simulink model "wlan_phy_tx_pmd"  (Simulink 7.8)
settings: Solver=VariableStepDiscrete  SolverMode=SingleTasking  StartTime=0.0  StopTime=inf  RelTol=1e-3
PostLoadFcn:
  | wlan_phy_tx_init
InitFcn:
  | wlan_phy_tx_init
StartFcn:
  | wlan_phy_tx_init
undefined symbols (not defined in the file): gcbh, ht_preamble_rom, MAX_CP_LEN, MAX_DATA_BITS_PER_SYM_PERIOD, MAX_NCBPS, MAX_NUM_BYTES, MAX_NUM_SC, MAX_NUM_SYMS, mcs_rom_11ag, mcs_rom_11n, Mod_Constellation_16QAM, Mod_Constellation_64QAM, Mod_Constellation_BPSK, Mod_Constellation_QPSK, Preamble_IQ, Preamble_IQ_scaled, tx_sim, wlan_tx_interleave_rom, xlBlockLoadCallback, xlGetNormalizedPeriod
libraries: xbsIndex_r4 x1358, xbsEDKLib_r4 x1
(part 9 of 10)

== system wlan_phy_tx_pmd/PSDU Syms Gen/Puncture & Interleave/Interleaver Ctrl & Puncturing/Interleave Mapping ==
  Base Rate Sym : Inport
  Ind A : Inport  Port=2
  Ind B : Inport  Port=3
  Concat1 : xbsIndex_r4/Concat  num_inputs=2  dbl_ovrd=off  block_type=concat
  Concat2 : xbsIndex_r4/Concat  num_inputs=3  dbl_ovrd=off  block_type=concat
  Concat3 : xbsIndex_r4/Concat  num_inputs=3  dbl_ovrd=off  block_type=concat
  Constant8 : xbsIndex_r4/Constant  const=0  gui_display_data_type=Fixed-point  arith_type=Unsigned  n_bits=ceil(log2(MAX_NCBPS))  bin_pt=0  preci_type=Single  exp_width=8  frac_width=24  explicit_period=off  period=1  equ=P=C  opselect=C  inp2=PCIN>>17  opr=+  inp1=P  carry=CIN  dbl_ovrd=off  block_type=constant
  Constant9 : xbsIndex_r4/Constant  const=0  gui_display_data_type=Boolean  arith_type=Boolean  n_bits=2  bin_pt=0  preci_type=Single  exp_width=8  frac_width=24  explicit_period=off  period=1  equ=P=C  opselect=C  inp2=PCIN>>17  opr=+  inp1=P  carry=CIN  dbl_ovrd=off  block_type=constant
  Inverter : xbsIndex_r4/Inverter  en=off  latency=0  dbl_ovrd=off  block_type=inv
  Logical : xbsIndex_r4/Logical  logical_function=AND  inputs=2  en=off  latency=0  precision=Full  arith_type=Unsigned  n_bits=16  bin_pt=0  align_bp=on  dbl_ovrd=off  block_type=logical
  Logical1 : xbsIndex_r4/Logical  logical_function=AND  inputs=2  en=off  latency=0  precision=Full  arith_type=Unsigned  n_bits=16  bin_pt=0  align_bp=on  dbl_ovrd=off  block_type=logical
  Map ROM : xbsIndex_r4/Dual Port RAM  depth=length(wlan_tx_interleave_rom)  initVector=wlan_tx_interleave_rom  distributed_mem=Block RAM  init_a=0  init_b=0  rst_a=off  rst_b=off  en_a=off  en_b=off  latency=1  write_mode_A=Read After Write  write_mode_B=Read After Write  dbl_ovrd=off  optimize=Area  block_type=dpram
  Addr A : Outport
  Addr B : Outport  Port=2
  wires:
  Base Rate Sym/1 -> Inverter/1
  Inverter/1 -> Logical/2, Concat1/1, Concat1/2
  Logical/1 -> Concat2/1, Concat3/1
  Logical1/1 -> Concat2/2, Concat3/2
  Ind A/1 -> Concat2/3
  [Tx_PHY_Mode_11n] -> Logical/1
  Concat2/1 -> Map ROM/1
  Ind B/1 -> Concat3/3
  Concat3/1 -> Map ROM/4
  Constant8/1 -> Map ROM/2, Map ROM/5
  Constant9/1 -> Map ROM/3, Map ROM/6
  Map ROM/1 -> Addr A/1
  Map ROM/2 -> Addr B/1
  [OFDM_TX_DATA_Mod_Sel] -> Logical1/2
  Concat1/1 -> Logical1/1

== system wlan_phy_tx_pmd/PSDU Syms Gen/Puncture & Interleave/Interleaver Ctrl & Puncturing/Puncturing ==
  Code Rate : Inport
  Reset : Inport  Port=2
  En : Inport  Port=3
  Inverter : xbsIndex_r4/Inverter  en=off  latency=0  dbl_ovrd=off  block_type=inv
  Inverter1 : xbsIndex_r4/Inverter  en=off  latency=0  dbl_ovrd=off  block_type=inv
  Logical : xbsIndex_r4/Logical  logical_function=AND  inputs=2  en=off  latency=0  precision=Full  arith_type=Unsigned  n_bits=16  bin_pt=0  align_bp=on  dbl_ovrd=off  block_type=logical
  Logical1 : xbsIndex_r4/Logical  logical_function=AND  inputs=2  en=off  latency=0  precision=Full  arith_type=Unsigned  n_bits=16  bin_pt=0  align_bp=on  dbl_ovrd=off  block_type=logical
  Mux1 : xbsIndex_r4/Mux  inputs=4  en=off  latency=0  precision=Full  arith_type=Unsigned  n_bits=16  bin_pt=14  quantization=Truncate  overflow=Wrap  dbl_ovrd=off  block_type=mux
  Mux3 : xbsIndex_r4/Mux  inputs=4  en=off  latency=0  precision=Full  arith_type=Unsigned  n_bits=16  bin_pt=14  quantization=Truncate  overflow=Wrap  dbl_ovrd=off  block_type=mux
  Mux4 : xbsIndex_r4/Mux  inputs=4  en=off  latency=0  precision=Full  arith_type=Unsigned  n_bits=16  bin_pt=14  quantization=Truncate  overflow=Wrap  dbl_ovrd=off  block_type=mux
  Rate 1/2 : Subsystem
  Rate 2/3 : Subsystem
  Rate 3/4 : Subsystem
  Rate 5/6 : Subsystem
  Index Inc : Outport
  Wr A : Outport  Port=2
  Wr B : Outport  Port=3
  wires:
  Mux3/1 -> Inverter/1
  Rate 1/2/1(Ind Inc) -> [R12_INC_A]
  Rate 1/2/2(Skip A) -> [R12_SKIP_A]
  Rate 1/2/3(Skip B) -> [R12_SKIP_B]
  Rate 2/3/1(Ind Inc) -> [R23_INC_A]
  Rate 2/3/2(Skip A) -> [R23_SKIP_A]
  Rate 2/3/3(Skip B) -> [R23_SKIP_B]
  Rate 3/4/1(Ind Inc) -> [R34_INC_A]
  Rate 3/4/2(Skip A) -> [R34_SKIP_A]
  Rate 3/4/3(Skip B) -> [R34_SKIP_B]
  [R12_SKIP_A] -> Mux3/2
  [R23_SKIP_A] -> Mux3/3
  [R34_SKIP_A] -> Mux3/4
  Mux1/1 -> Inverter1/1
  [R12_SKIP_B] -> Mux1/2
  [R23_SKIP_B] -> Mux1/3
  [R34_SKIP_B] -> Mux1/4
  [R12_INC_A] -> Mux4/2
  [R23_INC_A] -> Mux4/3
  [R34_INC_A] -> Mux4/4
  [R56_INC_A] -> Mux4/5
  [R56_SKIP_A] -> Mux3/5
  Rate 5/6/1(Ind Inc) -> [R56_INC_A]
  Rate 5/6/2(Skip A) -> [R56_SKIP_A]
  Rate 5/6/3(Skip B) -> [R56_SKIP_B]
  [R56_SKIP_B] -> Mux1/5
  Code Rate/1 -> Mux4/1, Mux3/1, Mux1/1
  Mux4/1 -> Index Inc/1
  Inverter/1 -> Logical/1
  Inverter1/1 -> Logical1/1
  Reset/1 -> Rate 1/2/1(Rst), Rate 2/3/1(Rst), Rate 3/4/1(Rst), Rate 5/6/1(Rst)
  En/1 -> Rate 1/2/2(En), Rate 2/3/2(En), Rate 3/4/2(En), Rate 5/6/2(En), Logical1/2, Logical/2
  Logical/1 -> Wr A/1
  Logical1/1 -> Wr B/1

== system wlan_phy_tx_pmd/PSDU Syms Gen/Puncture & Interleave/Interleaver Ctrl & Puncturing/negedge ==
  D : Inport
  Delay : xbsIndex_r4/Delay  rst=off  infoeditControl=Selection of Reset will increase slice count due to use of real FFs and instead of SRLs  en=off  latency=1  dbl_ovrd=off  reg_retiming=off  block_type=delay
      settings: infoedit=Hardware notes: A delay line is a chain, each link of which is an SRL16 followed by a flip-flop. If register retiming is enabled, the delay line is a chain of flip-flops.  xl_area=[1 1 0 0 0 0 0]  block_version=VER_STRING_GOES_HERE
  Inverter : xbsIndex_r4/Inverter  en=off  latency=0  dbl_ovrd=off  block_type=inv
      settings: xl_area=[0 0 0 0 0 0 0]  block_version=VER_STRING_GOES_HERE
  Logical1 : xbsIndex_r4/Logical  logical_function=AND  inputs=2  en=off  latency=0  precision=Full  arith_type=Unsigned  n_bits=8  bin_pt=2  align_bp=on  dbl_ovrd=off  block_type=logical
      settings: xl_area=[1 0 0 1 0 0 0]  block_version=VER_STRING_GOES_HERE
  Q : Outport
  wires:
  D/1 -> Delay/1, Inverter/1
  Logical1/1 -> Q/1
  Delay/1 -> Logical1/1
  Inverter/1 -> Logical1/2

== system wlan_phy_tx_pmd/PSDU Syms Gen/Puncture & Interleave/Mem Sel/S-R Latch1 ==
  S : Inport
  R : Inport  Port=2
  Constant1 : xbsIndex_r4/Constant  const=1  gui_display_data_type=Fixed-point  arith_type=Boolean  n_bits=1  bin_pt=0  preci_type=Single  exp_width=8  frac_width=24  explicit_period=off  period=1  equ=P=C  opselect=C  inp2=PCIN>>17  opr=+  inp1=P  carry=CIN  dbl_ovrd=off  block_type=constant
      settings: block_version=VER_STRING_GOES_HERE
  Convert1 : xbsIndex_r4/Convert  gui_display_data_type=Boolean  arith_type=Boolean  n_bits=1  bin_pt=0  float_type=Single  exp_bits=8  fraction_bits=24  quantization=Truncate  overflow=Wrap  en=off  latency=0  dbl_ovrd=off  pipeline=off  block_type=convert
  Convert2 : xbsIndex_r4/Convert  gui_display_data_type=Boolean  arith_type=Boolean  n_bits=1  bin_pt=0  float_type=Single  exp_bits=8  fraction_bits=24  quantization=Truncate  overflow=Wrap  en=off  latency=0  dbl_ovrd=off  pipeline=off  block_type=convert
  Register2 : xbsIndex_r4/Register  init=0  rst=on  en=on  dbl_ovrd=off  block_type=register
      settings: xl_area=[1 1 0 0 0 0 0]  block_version=VER_STRING_GOES_HERE
  Q : Outport
  wires:
  Convert2/1 -> Register2/3
  Convert1/1 -> Register2/2
  Constant1/1 -> Register2/1
  R/1 -> Convert1/1
  Register2/1 -> Q/1
  S/1 -> Convert2/1

== system wlan_phy_tx_pmd/Start Ctrl/Tx Active Debug Signal/Dly/S-R Latch1 ==
  S : Inport
  R : Inport  Port=2
  Constant1 : xbsIndex_r4/Constant  const=1  gui_display_data_type=Fixed-point  arith_type=Unsigned  n_bits=1  bin_pt=0  preci_type=Single  exp_width=8  frac_width=24  explicit_period=off  period=1  equ=P=C  opselect=C  inp2=PCIN>>17  opr=+  inp1=P  carry=CIN  dbl_ovrd=off  block_type=constant
      settings: block_version=VER_STRING_GOES_HERE
  Convert1 : xbsIndex_r4/Convert  gui_display_data_type=Boolean  arith_type=Boolean  n_bits=1  bin_pt=0  float_type=Single  exp_bits=8  fraction_bits=24  quantization=Truncate  overflow=Wrap  en=off  latency=0  dbl_ovrd=off  pipeline=off  block_type=convert
  Convert2 : xbsIndex_r4/Convert  gui_display_data_type=Boolean  arith_type=Boolean  n_bits=1  bin_pt=0  float_type=Single  exp_bits=8  fraction_bits=24  quantization=Truncate  overflow=Wrap  en=off  latency=0  dbl_ovrd=off  pipeline=off  block_type=convert
  Register2 : xbsIndex_r4/Register  init=0  rst=on  en=on  dbl_ovrd=off  block_type=register
      settings: xl_area=[1 1 0 0 0 0 0]  block_version=VER_STRING_GOES_HERE
  Q : Outport
  wires:
  Convert2/1 -> Register2/3
  Convert1/1 -> Register2/2
  Constant1/1 -> Register2/1
  R/1 -> Convert1/1
  Register2/1 -> Q/1
  S/1 -> Convert2/1

== system wlan_phy_tx_pmd/Start Ctrl/Tx Active Debug Signal/Dly/S-R Latch2 ==
  S : Inport
  R : Inport  Port=2
  Constant1 : xbsIndex_r4/Constant  const=1  gui_display_data_type=Fixed-point  arith_type=Unsigned  n_bits=1  bin_pt=0  preci_type=Single  exp_width=8  frac_width=24  explicit_period=off  period=1  equ=P=C  opselect=C  inp2=PCIN>>17  opr=+  inp1=P  carry=CIN  dbl_ovrd=off  block_type=constant
      settings: block_version=VER_STRING_GOES_HERE
  Convert1 : xbsIndex_r4/Convert  gui_display_data_type=Boolean  arith_type=Boolean  n_bits=1  bin_pt=0  float_type=Single  exp_bits=8  fraction_bits=24  quantization=Truncate  overflow=Wrap  en=off  latency=0  dbl_ovrd=off  pipeline=off  block_type=convert
  Convert2 : xbsIndex_r4/Convert  gui_display_data_type=Boolean  arith_type=Boolean  n_bits=1  bin_pt=0  float_type=Single  exp_bits=8  fraction_bits=24  quantization=Truncate  overflow=Wrap  en=off  latency=0  dbl_ovrd=off  pipeline=off  block_type=convert
  Register2 : xbsIndex_r4/Register  init=0  rst=on  en=on  dbl_ovrd=off  block_type=register
      settings: xl_area=[1 1 0 0 0 0 0]  block_version=VER_STRING_GOES_HERE
  Q : Outport
  wires:
  S/1 -> Convert2/1
  Register2/1 -> Q/1
  R/1 -> Convert1/1
  Constant1/1 -> Register2/1
  Convert1/1 -> Register2/2
  Convert2/1 -> Register2/3

== system wlan_phy_tx_pmd/PSDU Syms Gen/Modulate/Control & Pilots/Pilot Gen/Pilot Selection ==
  note: All PHY modes:
      | -Pilot tones in subcarriers [-21,-7,7,21]
      | -Subcarriers [-7,-21] are x_ind [57,43]
      | -One pilot per OFDM sybmol is opposite sign of other 3
      |
      | 11a/g:
      | -Opposite sign always in subcarrier 21
      |
      | 11n/ac:
      | -Syms 0:4: Same as a/g
      | -Syms 5:6: No pilot tones in HT-STF, HT-LTF
      | -Syms 7:N: Opposite sign pilot rotates across 4 subcarriers sequentially:
      |    7: 21
      |    8: 7
      |    9: -21
      |    10: -7
      |     ...
      | Logic uses 2LSB of sym index to select current negative pilot subcarrier
  sc_ind : Inport
  Shift : Inport  Port=2
  Constant1 : xbsIndex_r4/Constant  const=21  gui_display_data_type=Fixed-point  arith_type=Unsigned  n_bits=6  bin_pt=0  preci_type=Single  exp_width=8  frac_width=24  explicit_period=off  period=8  equ=P=C  opselect=C  inp2=PCIN>>17  opr=+  inp1=P  carry=CIN  dbl_ovrd=off  block_type=constant
  Constant2 : xbsIndex_r4/Constant  const=7  gui_display_data_type=Fixed-point  arith_type=Unsigned  n_bits=6  bin_pt=0  preci_type=Single  exp_width=8  frac_width=24  explicit_period=off  period=8  equ=P=C  opselect=C  inp2=PCIN>>17  opr=+  inp1=P  carry=CIN  dbl_ovrd=off  block_type=constant
  Constant3 : xbsIndex_r4/Constant  const=64-7  gui_display_data_type=Fixed-point  arith_type=Unsigned  n_bits=6  bin_pt=0  preci_type=Single  exp_width=8  frac_width=24  explicit_period=off  period=8  equ=P=C  opselect=C  inp2=PCIN>>17  opr=+  inp1=P  carry=CIN  dbl_ovrd=off  block_type=constant
  Constant4 : xbsIndex_r4/Constant  const=64-21  gui_display_data_type=Fixed-point  arith_type=Unsigned  n_bits=6  bin_pt=0  preci_type=Single  exp_width=8  frac_width=24  explicit_period=off  period=8  equ=P=C  opselect=C  inp2=PCIN>>17  opr=+  inp1=P  carry=CIN  dbl_ovrd=off  block_type=constant
  Logical1 : xbsIndex_r4/Logical  logical_function=OR  inputs=4  en=off  latency=0  precision=Full  arith_type=Unsigned  n_bits=8  bin_pt=2  align_bp=on  dbl_ovrd=off  block_type=logical
      settings: xl_area=[2 0 0 2 0 0 0]  block_version=VER_STRING_GOES_HERE
  Mux : xbsIndex_r4/Mux  inputs=4  en=off  latency=0  precision=Full  arith_type=Unsigned  n_bits=16  bin_pt=14  quantization=Truncate  overflow=Wrap  dbl_ovrd=off  block_type=mux
  Relational{4..7} (4 alike) : xbsIndex_r4/Relational  mode=a=b  en=off  latency=0  dbl_ovrd=off  block_type=relational
      settings: xl_area=[2 0 0 3 0 0 0]  block_version=VER_STRING_GOES_HERE
  Pilot : Outport
  Negate : Outport  Port=2
  wires:
  Constant1/1 -> Relational5/1
  Constant2/1 -> Relational4/1
  Relational4/1 -> Logical1/1, Mux/3
  Relational5/1 -> Mux/2, Logical1/2
  Relational6/1 -> Logical1/3, Mux/5
  Relational7/1 -> Logical1/4, Mux/4
  sc_ind/1 -> Relational4/2, Relational5/2, Relational6/2, Relational7/2
  Logical1/1 -> Pilot/1
  Constant4/1 -> Relational6/1
  Constant3/1 -> Relational7/1
  Mux/1 -> Negate/1
  Shift/1 -> Mux/1

== system wlan_phy_tx_pmd/PSDU Syms Gen/Modulate/Control & Pilots/Pilot Gen/Posedge ==
  note: Rising Edge Detection
  D : Inport
  Delay : xbsIndex_r4/Delay  rst=off  infoeditControl=Selection of Reset will increase slice count due to use of real FFs and instead of SRLs  en=off  latency=1  dbl_ovrd=off  reg_retiming=off  block_type=delay
      settings: infoedit=Hardware notes: A delay line is a chain, each link of which is an SRL16 followed by a flip-flop. If register retiming is enabled, the delay line is a chain of flip-flops.  xl_area=[1 1 0 0 0 0 0]  block_version=VER_STRING_GOES_HERE
  Inverter : xbsIndex_r4/Inverter  en=off  latency=0  dbl_ovrd=off  block_type=inv
      settings: xl_area=[0 0 0 0 0 0 0]  block_version=VER_STRING_GOES_HERE
  Logical1 : xbsIndex_r4/Logical  logical_function=AND  inputs=2  en=off  latency=0  precision=Full  arith_type=Unsigned  n_bits=8  bin_pt=2  align_bp=on  dbl_ovrd=off  block_type=logical
      settings: xl_area=[1 0 0 1 0 0 0]  block_version=VER_STRING_GOES_HERE
  Q : Outport
  wires:
  D/1 -> Logical1/2, Delay/1
  Logical1/1 -> Q/1
  Inverter/1 -> Logical1/1
  Delay/1 -> Inverter/1

== system wlan_phy_tx_pmd/PSDU Syms Gen/Modulate/Control & Pilots/Pilot Gen/Scrambling LFSR ==
  en : Inport
  rst : Inport  Port=2
  Assert : xbsIndex_r4/Assert  assert_type=on  type_source=Explicitly  gui_display_data_type=Boolean  arith_type=Boolean  n_bits=16  bin_pt=14  preci_type=Single  exp_width=8  frac_width=24  assert_rate=on  rate_source=Explicitly  period=1  output_port=on  block_type=assert
      settings: block_version=VER_STRING_GOES_HERE
  Assert1 : xbsIndex_r4/Assert  assert_type=on  type_source=Explicitly  gui_display_data_type=Fixed-point  arith_type=Boolean  n_bits=16  bin_pt=14  preci_type=Single  exp_width=8  frac_width=24  assert_rate=on  rate_source=Explicitly  period=1  output_port=on  block_type=assert
      settings: infoedit=Asserts a user-defined sample rate and/or type on a signal.<P><P>Hardware notes: In hardware this block costs nothing.  block_version=VER_STRING_GOES_HERE
  Convert : xbsIndex_r4/Convert  gui_display_data_type=Boolean  arith_type=Boolean  n_bits=16  bin_pt=14  float_type=Single  exp_bits=8  fraction_bits=24  quantization=Truncate  overflow=Wrap  en=off  latency=0  dbl_ovrd=off  pipeline=off  block_type=convert
  Convert1 : xbsIndex_r4/Convert  gui_display_data_type=Boolean  arith_type=Boolean  n_bits=16  bin_pt=14  float_type=Single  exp_bits=8  fraction_bits=24  quantization=Truncate  overflow=Wrap  en=off  latency=0  dbl_ovrd=off  pipeline=off  block_type=convert
  Logical : xbsIndex_r4/Logical  logical_function=XOR  inputs=2  en=off  latency=0  precision=Full  arith_type=Unsigned  n_bits=8  bin_pt=2  align_bp=on  dbl_ovrd=off  block_type=logical
      settings: xl_area=[0, 0, 0, 0, 0, 0, 0]  block_version=VER_STRING_GOES_HERE
  Register{,1..6} (7 alike) : xbsIndex_r4/Register  init=1  rst=on  en=on  dbl_ovrd=off  block_type=register
      settings: xl_area=[0, 0, 0, 0, 0, 0, 0]  block_version=VER_STRING_GOES_HERE
  Q : Outport
  wires:
  rst/1 -> Convert/1
  Register6/1 -> Assert/1
  Logical/1 -> Register/1, Q/1
  Register5/1 -> Register6/1
  Register4/1 -> Register5/1
  Register3/1 -> Register4/1, Assert1/1
  Register2/1 -> Register3/1
  Register1/1 -> Register2/1
  Register/1 -> Register1/1
  Assert/1 -> Logical/1
  Assert1/1 -> Logical/2
  en/1 -> Convert1/1
  Convert/1 -> Register/2, Register1/2, Register2/2, Register3/2, Register4/2, Register5/2, Register6/2
  Convert1/1 -> Register/3, Register1/3, Register2/3, Register3/3, Register4/3, Register5/3, Register6/3

== system wlan_phy_tx_pmd/PSDU Syms Gen/Pkt Data/BRAM IF 64b/BRAM Interface/Sim RAM ==
  note: This subsystem is only used in simulation.
      |
      | The ROMs below emulate the Tx packet buffer in the full 802.11 Reference Design.
      | These ROMs are initalized with a packet defined in the .m init script. The PHY uses
      | this packet in its simulation. In hardware the PHY pulls its packets directly from
      | the Tx packet buffer, whose contents are controlled by the MAC software.
      |
      | These ROMs accurately mimic the 1 cycle latency for accessing the packet buffer BRAMs
      | in the real design. It is essential the packet buffer implementation honor this 1-cycle
      | assumption.
  Addr : Inport
  Concat : xbsIndex_r4/Concat  num_inputs=2  dbl_ovrd=off  block_type=concat
  Convert2 : xbsIndex_r4/Convert  gui_display_data_type=Fixed-point  arith_type=Unsigned  n_bits=ceil(log2(MAX_NUM_BYTES))-3  bin_pt=0  float_type=Single  exp_bits=8  fraction_bits=24  quantization=Truncate  overflow=Wrap  en=off  latency=0  dbl_ovrd=off  pipeline=off  block_type=convert
  Disregard Subsystem : xbsIndex_r4/Disregard Subsystem  Tag=discardX  block_type=disregard
  ROM1 : xbsIndex_r4/ROM  depth=MAX_NUM_BYTES/8  initVector=PPDU_words(2:2:end)  distributed_mem=Block RAM  rst=off  init_reg=0  en=off  latency=1  gui_display_data_type=Fixed-point  arith_type=Unsigned  n_bits=32  bin_pt=0  preci_type=Single  exp_width=8  frac_width=24  dbl_ovrd=off  optimize=Area  use_rpm=on  block_type=sprom
  ROM2 : xbsIndex_r4/ROM  depth=MAX_NUM_BYTES/8  initVector=PPDU_words(1:2:end)  distributed_mem=Block RAM  rst=off  init_reg=0  en=off  latency=1  gui_display_data_type=Fixed-point  arith_type=Unsigned  n_bits=32  bin_pt=0  preci_type=Single  exp_width=8  frac_width=24  dbl_ovrd=off  optimize=Area  use_rpm=on  block_type=sprom
  64b : Outport
  wires:
  Concat/1 -> 64b/1
  ROM1/1 -> Concat/1
  ROM2/1 -> Concat/2
  Convert2/1 -> ROM1/1, ROM2/1
  Addr/1 -> Convert2/1

== system wlan_phy_tx_pmd/PSDU Syms Gen/Pkt Data/FCS Calc/CRC32 Calc/Endian Swap ==
  B : Inport
  Concat : xbsIndex_r4/Concat  num_inputs=8  dbl_ovrd=off  block_type=concat
  b0 : xbsIndex_r4/Slice  nbits=1  boolean_output=off  mode=Lower Bit Location + Width  bit1=0  base1=MSB of Input  bit0=0  base0=LSB of Input  dbl_ovrd=off  block_type=slice
  b1 : xbsIndex_r4/Slice  nbits=1  boolean_output=off  mode=Lower Bit Location + Width  bit1=0  base1=MSB of Input  bit0=1  base0=LSB of Input  dbl_ovrd=off  block_type=slice
  b2 : xbsIndex_r4/Slice  nbits=1  boolean_output=off  mode=Lower Bit Location + Width  bit1=0  base1=MSB of Input  bit0=2  base0=LSB of Input  dbl_ovrd=off  block_type=slice
  b3 : xbsIndex_r4/Slice  nbits=1  boolean_output=off  mode=Lower Bit Location + Width  bit1=0  base1=MSB of Input  bit0=3  base0=LSB of Input  dbl_ovrd=off  block_type=slice
  b4 : xbsIndex_r4/Slice  nbits=1  boolean_output=off  mode=Lower Bit Location + Width  bit1=0  base1=MSB of Input  bit0=4  base0=LSB of Input  dbl_ovrd=off  block_type=slice
  b5 : xbsIndex_r4/Slice  nbits=1  boolean_output=off  mode=Lower Bit Location + Width  bit1=0  base1=MSB of Input  bit0=5  base0=LSB of Input  dbl_ovrd=off  block_type=slice
  b6 : xbsIndex_r4/Slice  nbits=1  boolean_output=off  mode=Lower Bit Location + Width  bit1=0  base1=MSB of Input  bit0=6  base0=LSB of Input  dbl_ovrd=off  block_type=slice
  b7 : xbsIndex_r4/Slice  nbits=1  boolean_output=off  mode=Lower Bit Location + Width  bit1=0  base1=MSB of Input  bit0=7  base0=LSB of Input  dbl_ovrd=off  block_type=slice
  I : Outport
  wires:
  b7/1 -> Concat/8
  Concat/1 -> I/1
  b6/1 -> Concat/7
  b5/1 -> Concat/6
  b4/1 -> Concat/5
  b3/1 -> Concat/4
  b2/1 -> Concat/3
  b1/1 -> Concat/2
  b0/1 -> Concat/1
  B/1 -> b7/1, b6/1, b5/1, b4/1, b3/1, b2/1, b1/1, b0/1

== system wlan_phy_tx_pmd/PSDU Syms Gen/Pkt Data/FCS Calc/CRC32 Calc/Endian Swap1 ==
  B : Inport
  Concat : xbsIndex_r4/Concat  num_inputs=8  dbl_ovrd=off  block_type=concat
  b0 : xbsIndex_r4/Slice  nbits=1  boolean_output=off  mode=Lower Bit Location + Width  bit1=0  base1=MSB of Input  bit0=0  base0=LSB of Input  dbl_ovrd=off  block_type=slice
  b1 : xbsIndex_r4/Slice  nbits=1  boolean_output=off  mode=Lower Bit Location + Width  bit1=0  base1=MSB of Input  bit0=1  base0=LSB of Input  dbl_ovrd=off  block_type=slice
  b2 : xbsIndex_r4/Slice  nbits=1  boolean_output=off  mode=Lower Bit Location + Width  bit1=0  base1=MSB of Input  bit0=2  base0=LSB of Input  dbl_ovrd=off  block_type=slice
  b3 : xbsIndex_r4/Slice  nbits=1  boolean_output=off  mode=Lower Bit Location + Width  bit1=0  base1=MSB of Input  bit0=3  base0=LSB of Input  dbl_ovrd=off  block_type=slice
  b4 : xbsIndex_r4/Slice  nbits=1  boolean_output=off  mode=Lower Bit Location + Width  bit1=0  base1=MSB of Input  bit0=4  base0=LSB of Input  dbl_ovrd=off  block_type=slice
  b5 : xbsIndex_r4/Slice  nbits=1  boolean_output=off  mode=Lower Bit Location + Width  bit1=0  base1=MSB of Input  bit0=5  base0=LSB of Input  dbl_ovrd=off  block_type=slice
  b6 : xbsIndex_r4/Slice  nbits=1  boolean_output=off  mode=Lower Bit Location + Width  bit1=0  base1=MSB of Input  bit0=6  base0=LSB of Input  dbl_ovrd=off  block_type=slice
  b7 : xbsIndex_r4/Slice  nbits=1  boolean_output=off  mode=Lower Bit Location + Width  bit1=0  base1=MSB of Input  bit0=7  base0=LSB of Input  dbl_ovrd=off  block_type=slice
  I : Outport
  wires:
  B/1 -> b0/1, b1/1, b2/1, b3/1, b4/1, b5/1, b6/1, b7/1
  b0/1 -> Concat/1
  b1/1 -> Concat/2
  b2/1 -> Concat/3
  b3/1 -> Concat/4
  b4/1 -> Concat/5
  b5/1 -> Concat/6
  b6/1 -> Concat/7
  Concat/1 -> I/1
  b7/1 -> Concat/8

== system wlan_phy_tx_pmd/PSDU Syms Gen/Pkt Data/FCS Calc/CRC32 Calc/Endian Swap2 ==
  B : Inport
  Concat : xbsIndex_r4/Concat  num_inputs=8  dbl_ovrd=off  block_type=concat
  b0 : xbsIndex_r4/Slice  nbits=1  boolean_output=off  mode=Lower Bit Location + Width  bit1=0  base1=MSB of Input  bit0=0  base0=LSB of Input  dbl_ovrd=off  block_type=slice
  b1 : xbsIndex_r4/Slice  nbits=1  boolean_output=off  mode=Lower Bit Location + Width  bit1=0  base1=MSB of Input  bit0=1  base0=LSB of Input  dbl_ovrd=off  block_type=slice
  b2 : xbsIndex_r4/Slice  nbits=1  boolean_output=off  mode=Lower Bit Location + Width  bit1=0  base1=MSB of Input  bit0=2  base0=LSB of Input  dbl_ovrd=off  block_type=slice
  b3 : xbsIndex_r4/Slice  nbits=1  boolean_output=off  mode=Lower Bit Location + Width  bit1=0  base1=MSB of Input  bit0=3  base0=LSB of Input  dbl_ovrd=off  block_type=slice
  b4 : xbsIndex_r4/Slice  nbits=1  boolean_output=off  mode=Lower Bit Location + Width  bit1=0  base1=MSB of Input  bit0=4  base0=LSB of Input  dbl_ovrd=off  block_type=slice
  b5 : xbsIndex_r4/Slice  nbits=1  boolean_output=off  mode=Lower Bit Location + Width  bit1=0  base1=MSB of Input  bit0=5  base0=LSB of Input  dbl_ovrd=off  block_type=slice
  b6 : xbsIndex_r4/Slice  nbits=1  boolean_output=off  mode=Lower Bit Location + Width  bit1=0  base1=MSB of Input  bit0=6  base0=LSB of Input  dbl_ovrd=off  block_type=slice
  b7 : xbsIndex_r4/Slice  nbits=1  boolean_output=off  mode=Lower Bit Location + Width  bit1=0  base1=MSB of Input  bit0=7  base0=LSB of Input  dbl_ovrd=off  block_type=slice
  I : Outport
  wires:
  b7/1 -> Concat/8
  Concat/1 -> I/1
  b6/1 -> Concat/7
  b5/1 -> Concat/6
  b4/1 -> Concat/5
  b3/1 -> Concat/4
  b2/1 -> Concat/3
  b1/1 -> Concat/2
  b0/1 -> Concat/1
  B/1 -> b7/1, b6/1, b5/1, b4/1, b3/1, b2/1, b1/1, b0/1

== system wlan_phy_tx_pmd/PSDU Syms Gen/Pkt Data/FCS Calc/CRC32 Calc/Endian Swap3 ==
  B : Inport
  Concat : xbsIndex_r4/Concat  num_inputs=8  dbl_ovrd=off  block_type=concat
  b0 : xbsIndex_r4/Slice  nbits=1  boolean_output=off  mode=Lower Bit Location + Width  bit1=0  base1=MSB of Input  bit0=0  base0=LSB of Input  dbl_ovrd=off  block_type=slice
  b1 : xbsIndex_r4/Slice  nbits=1  boolean_output=off  mode=Lower Bit Location + Width  bit1=0  base1=MSB of Input  bit0=1  base0=LSB of Input  dbl_ovrd=off  block_type=slice
  b2 : xbsIndex_r4/Slice  nbits=1  boolean_output=off  mode=Lower Bit Location + Width  bit1=0  base1=MSB of Input  bit0=2  base0=LSB of Input  dbl_ovrd=off  block_type=slice
  b3 : xbsIndex_r4/Slice  nbits=1  boolean_output=off  mode=Lower Bit Location + Width  bit1=0  base1=MSB of Input  bit0=3  base0=LSB of Input  dbl_ovrd=off  block_type=slice
  b4 : xbsIndex_r4/Slice  nbits=1  boolean_output=off  mode=Lower Bit Location + Width  bit1=0  base1=MSB of Input  bit0=4  base0=LSB of Input  dbl_ovrd=off  block_type=slice
  b5 : xbsIndex_r4/Slice  nbits=1  boolean_output=off  mode=Lower Bit Location + Width  bit1=0  base1=MSB of Input  bit0=5  base0=LSB of Input  dbl_ovrd=off  block_type=slice
  b6 : xbsIndex_r4/Slice  nbits=1  boolean_output=off  mode=Lower Bit Location + Width  bit1=0  base1=MSB of Input  bit0=6  base0=LSB of Input  dbl_ovrd=off  block_type=slice
  b7 : xbsIndex_r4/Slice  nbits=1  boolean_output=off  mode=Lower Bit Location + Width  bit1=0  base1=MSB of Input  bit0=7  base0=LSB of Input  dbl_ovrd=off  block_type=slice
  I : Outport
  wires:
  B/1 -> b0/1, b1/1, b2/1, b3/1, b4/1, b5/1, b6/1, b7/1
  b0/1 -> Concat/1
  b1/1 -> Concat/2
  b2/1 -> Concat/3
  b3/1 -> Concat/4
  b4/1 -> Concat/5
  b5/1 -> Concat/6
  b6/1 -> Concat/7
  Concat/1 -> I/1
  b7/1 -> Concat/8

== system wlan_phy_tx_pmd/PSDU Syms Gen/Pkt Data/FCS Calc/CRC32 Calc/Endian Swap4 ==
  B : Inport
  Concat : xbsIndex_r4/Concat  num_inputs=8  dbl_ovrd=off  block_type=concat
  b0 : xbsIndex_r4/Slice  nbits=1  boolean_output=off  mode=Lower Bit Location + Width  bit1=0  base1=MSB of Input  bit0=0  base0=LSB of Input  dbl_ovrd=off  block_type=slice
  b1 : xbsIndex_r4/Slice  nbits=1  boolean_output=off  mode=Lower Bit Location + Width  bit1=0  base1=MSB of Input  bit0=1  base0=LSB of Input  dbl_ovrd=off  block_type=slice
  b2 : xbsIndex_r4/Slice  nbits=1  boolean_output=off  mode=Lower Bit Location + Width  bit1=0  base1=MSB of Input  bit0=2  base0=LSB of Input  dbl_ovrd=off  block_type=slice
  b3 : xbsIndex_r4/Slice  nbits=1  boolean_output=off  mode=Lower Bit Location + Width  bit1=0  base1=MSB of Input  bit0=3  base0=LSB of Input  dbl_ovrd=off  block_type=slice
  b4 : xbsIndex_r4/Slice  nbits=1  boolean_output=off  mode=Lower Bit Location + Width  bit1=0  base1=MSB of Input  bit0=4  base0=LSB of Input  dbl_ovrd=off  block_type=slice
  b5 : xbsIndex_r4/Slice  nbits=1  boolean_output=off  mode=Lower Bit Location + Width  bit1=0  base1=MSB of Input  bit0=5  base0=LSB of Input  dbl_ovrd=off  block_type=slice
  b6 : xbsIndex_r4/Slice  nbits=1  boolean_output=off  mode=Lower Bit Location + Width  bit1=0  base1=MSB of Input  bit0=6  base0=LSB of Input  dbl_ovrd=off  block_type=slice
  b7 : xbsIndex_r4/Slice  nbits=1  boolean_output=off  mode=Lower Bit Location + Width  bit1=0  base1=MSB of Input  bit0=7  base0=LSB of Input  dbl_ovrd=off  block_type=slice
  I : Outport
  wires:
  b7/1 -> Concat/8
  Concat/1 -> I/1
  b6/1 -> Concat/7
  b5/1 -> Concat/6
  b4/1 -> Concat/5
  b3/1 -> Concat/4
  b2/1 -> Concat/3
  b1/1 -> Concat/2
  b0/1 -> Concat/1
  B/1 -> b7/1, b6/1, b5/1, b4/1, b3/1, b2/1, b1/1, b0/1

== system wlan_phy_tx_pmd/PSDU Syms Gen/Pkt Data/SIGNAL & HT-SIG Decode/HT-SIG Decode/CRC8 Calc ==
  note: This logic implements parallel version of the 8-bit shift register shown in IEEE 802.11-2012 20.3.9.4.4. The crc_accum
      | block contains the shift register state after the first 4 bytes of the HT-SIG are read. The CRC value must then be updated by
      | loading 2 additional 0 bits (the N_ESS bits) to comptue the final CRC value used as the 8-bit checksum in the HT-SIG field.
      |
      | Given the state of the shift register after loading 32 message bits, it is possible to directly compute the final shift register state.
      |
      | Let C[7:0] be value of CRC shift register (crc_accum here) after first 32 bits (4 bytes) have been processed.
      |
      | Assume 2LSB of byte 4, NUM_ESS in the HT-SIG defintion, are 00. This is definitely true for this version of the Tx PHY.
      |
      | Final 8-bit checksum value can be computed by initializing the CRC shift register with C[7:0], then shifting in two zero message bits.
      |
      | The shift register state after loading 1 zero message bit (Cb1[7:0]) as a function of C:
      |
      | Cb1[7:3] = C[6:2]
      | Cb1[  2] = C[1] ^ C[7]
      | Cb1[  1] = C[0] ^ C[7]
      | Cb1[  0] = C[7]
      |
      | The final state of the shift register CF[7:0] can be expressed as a function of Cb1:
      |
      | CF[7:3] = Cb1[6:2]
      | CF[  2] = Cb1[1] ^ Cb1[7]
      | CF[  1] = Cb1[0] ^ Cb1[7]
      | CF[  0] = Cb1[7]
      |
      | Expanding Cb1 gives CF as a function of C:
      |
      | CF[7:4] = C[5:2]               (== Cb1[6:3])
      | CF[  3] = C[1] ^ C[7]          (== Cb1[2])
      | CF[  2] = C[0] ^ C[7] ^ C[6]   (== Cb1[1] ^ Cb1[7])
      | CF[  1] = C[7] ^ C[6]          (== Cb1[0] ^ Cb1[7])
      | CF[  0] = C[6]                 (== Cb1[7])
  byte_ind : Inport
  data_valid : Inport  Port=2
  data_byte : Inport  Port=3
  reset : Inport  Port=4
  4LSB Calc : Subsystem
  Assert1 : xbsIndex_r4/Assert  assert_type=off  type_source=Explicitly  gui_display_data_type=Fixed-point  arith_type="Signed  (2's comp)"  n_bits=16  bin_pt=14  preci_type=Single  exp_width=8  frac_width=24  assert_rate=on  rate_source=Explicitly  period=1  output_port=on  block_type=assert
      settings: block_version=VER_STRING_GOES_HERE
  CRC8 Lookup : xbsIndex_r4/ROM  depth=256  initVector=CRC_Table8  distributed_mem=Distributed memory  rst=off  init_reg=0  en=off  latency=0  gui_display_data_type=Fixed-point  arith_type=Unsigned  n_bits=8  bin_pt=0  preci_type=Single  exp_width=8  frac_width=24  dbl_ovrd=off  optimize=Area  use_rpm=off  block_type=sprom
      settings: xl_area=[0, 0, 0, 0, 0, 0, 0]  block_version=VER_STRING_GOES_HERE
  Concat3 : xbsIndex_r4/Concat  num_inputs=2  dbl_ovrd=off  block_type=concat
  Constant3 : xbsIndex_r4/Constant  const=3  gui_display_data_type=Fixed-point  arith_type=Unsigned  n_bits=4  bin_pt=0  preci_type=Single  exp_width=8  frac_width=24  explicit_period=off  period=1  equ=P=C  opselect=C  inp2=PCIN>>17  opr=+  inp1=P  carry=CIN  dbl_ovrd=off  block_type=constant
  Constant4 : xbsIndex_r4/Constant  const=6  gui_display_data_type=Fixed-point  arith_type=Unsigned  n_bits=4  bin_pt=0  preci_type=Single  exp_width=8  frac_width=24  explicit_period=off  period=1  equ=P=C  opselect=C  inp2=PCIN>>17  opr=+  inp1=P  carry=CIN  dbl_ovrd=off  block_type=constant
  Endian Swap : Subsystem
  Inverter : xbsIndex_r4/Inverter  en=off  latency=0  dbl_ovrd=off  block_type=inv
  Logical1 : xbsIndex_r4/Logical  logical_function=AND  inputs=3  en=off  latency=0  precision=Full  arith_type=Unsigned  n_bits=16  bin_pt=0  align_bp=on  dbl_ovrd=off  block_type=logical
  Logical3 : xbsIndex_r4/Logical  logical_function=XOR  inputs=2  en=off  latency=0  precision=Full  arith_type=Unsigned  n_bits=8  bin_pt=2  align_bp=on  dbl_ovrd=off  block_type=logical
      settings: xl_area=[0, 0, 0, 0, 0, 0, 0]  block_version=VER_STRING_GOES_HERE
  Relational3 : xbsIndex_r4/Relational  mode=a>=b  en=off  latency=0  dbl_ovrd=off  block_type=relational
  Relational4 : xbsIndex_r4/Relational  mode=a<=b  en=off  latency=0  dbl_ovrd=off  block_type=relational
  b[5:2] : xbsIndex_r4/Slice  nbits=4  boolean_output=off  mode=Lower Bit Location + Width  bit1=0  base1=MSB of Input  bit0=2  base0=LSB of Input  dbl_ovrd=off  block_type=slice
  crc_accum : xbsIndex_r4/Register  init=hex2dec('FF')  rst=on  en=on  dbl_ovrd=off  block_type=register
      settings: xl_area=[0, 0, 0, 0, 0, 0, 0]  block_version=VER_STRING_GOES_HERE
  CRC8 : Outport
  wires:
  Endian Swap/1(I) -> Logical3/2
  CRC8 Lookup/1 -> crc_accum/1
  Assert1/1 -> Logical3/1, b[5:2]/1
  crc_accum/1 -> Assert1/1, 4LSB Calc/1(crc_accum)
  Logical3/1 -> CRC8 Lookup/1
  data_byte/1 -> Endian Swap/1(B)
  byte_ind/1 -> Relational4/1, Relational3/1
  Constant3/1 -> Relational3/2
  Constant4/1 -> Relational4/2
  data_valid/1 -> Logical1/1
  Relational3/1 -> Logical1/2
  Relational4/1 -> Logical1/3
  Logical1/1 -> crc_accum/3
  reset/1 -> crc_accum/2
  b[5:2]/1 -> Concat3/1
  4LSB Calc/1(Final 4LSB) -> Concat3/2
  Concat3/1 -> Inverter/1
  Inverter/1 -> CRC8/1

== system wlan_phy_tx_pmd/PSDU Syms Gen/Pkt Data/SIGNAL & HT-SIG Decode/HT-SIG Decode/Format ==
  note: Let checksum byte be C[7:0]
      | B5[7:0] = [0 0 0 0 0 0 C[0] C[1]]
      | B4[7:0] = [C[2] C[3] C[4] C[5] C[6] C[7] 0 0]
  CRC : Inport
  Concat1 : xbsIndex_r4/Concat  num_inputs=2  dbl_ovrd=off  block_type=concat
  Concat2 : xbsIndex_r4/Concat  num_inputs=2  dbl_ovrd=off  block_type=concat
  Constant1 : xbsIndex_r4/Constant  const=0  gui_display_data_type=Fixed-point  arith_type=Unsigned  n_bits=2  bin_pt=0  preci_type=Single  exp_width=8  frac_width=24  explicit_period=off  period=1  equ=P=C  opselect=C  inp2=PCIN>>17  opr=+  inp1=P  carry=CIN  dbl_ovrd=off  block_type=constant
  Constant2 : xbsIndex_r4/Constant  const=0  gui_display_data_type=Fixed-point  arith_type=Unsigned  n_bits=6  bin_pt=0  preci_type=Single  exp_width=8  frac_width=24  explicit_period=off  period=1  equ=P=C  opselect=C  inp2=PCIN>>17  opr=+  inp1=P  carry=CIN  dbl_ovrd=off  block_type=constant
  Endian Swap1 : Subsystem
  Endian Swap2 : Subsystem
  b[1:0] : xbsIndex_r4/Slice  nbits=2  boolean_output=off  mode=Lower Bit Location + Width  bit1=0  base1=MSB of Input  bit0=0  base0=LSB of Input  dbl_ovrd=off  block_type=slice
  b[7:2] : xbsIndex_r4/Slice  nbits=6  boolean_output=off  mode=Lower Bit Location + Width  bit1=0  base1=MSB of Input  bit0=2  base0=LSB of Input  dbl_ovrd=off  block_type=slice
  HTSIG[4] : Outport
  HTSIG[5] : Outport  Port=2
  wires:
  CRC/1 -> b[1:0]/1, b[7:2]/1
  Constant2/1 -> Concat1/2
  Endian Swap2/1(I) -> HTSIG[5]/1
  Endian Swap1/1(I) -> HTSIG[4]/1
  b[1:0]/1 -> Concat1/1
  Concat1/1 -> Endian Swap2/1(B)
  Constant1/1 -> Concat2/1
  b[7:2]/1 -> Concat2/2
  Concat2/1 -> Endian Swap1/1(B)

== system wlan_phy_tx_pmd/PSDU Syms Gen/Pkt Data/SIGNAL & HT-SIG Decode/HT-SIG Decode/HT Length ==
  B4 : Inport
  B5 : Inport  Port=2
  Concat1 : xbsIndex_r4/Concat  num_inputs=2  dbl_ovrd=off  block_type=concat
  length : Outport
  wires:
  B5/1 -> Concat1/1
  B4/1 -> Concat1/2
  Concat1/1 -> length/1

== system wlan_phy_tx_pmd/PSDU Syms Gen/Pkt Data/SIGNAL & HT-SIG Decode/HT-SIG Decode/HT-SIG Flags ==
  note: HT-SIG Flags
      | (IEEE 802.11-2012 Figured 20-6)
      |
      | B3[7]: Channel bandwidth (0=20, 1=40)
      |
      | B6[0]: Smoothing
      | B6[1]: Not sounding
      | B6[2]: Reserved (always 1)
      | B6[3]: Aggregation
      | B6[5:4]: STBC
      | B6[6]: FEC (0=BCC, 1=LDPC)
      | B6[7]: Short GI
      |
      | B7[1:0]: Num extension spatial streams
  B3 : Inport
  B6 : Inport  Port=2
  B7 : Inport  Port=3
  Constant : xbsIndex_r4/Constant  const=0  gui_display_data_type=Fixed-point  arith_type=Unsigned  n_bits=1  bin_pt=0  preci_type=Single  exp_width=8  frac_width=24  explicit_period=off  period=1  equ=P=C  opselect=C  inp2=PCIN>>17  opr=+  inp1=P  carry=CIN  dbl_ovrd=off  block_type=constant
  Constant1 : xbsIndex_r4/Constant  const=0  gui_display_data_type=Fixed-point  arith_type=Unsigned  n_bits=1  bin_pt=0  preci_type=Single  exp_width=8  frac_width=24  explicit_period=off  period=1  equ=P=C  opselect=C  inp2=PCIN>>17  opr=+  inp1=P  carry=CIN  dbl_ovrd=off  block_type=constant
  Logical : xbsIndex_r4/Logical  logical_function=OR  inputs=5  en=off  latency=0  precision=Full  arith_type=Unsigned  n_bits=16  bin_pt=0  align_bp=on  dbl_ovrd=off  block_type=logical
  Relational : xbsIndex_r4/Relational  mode=a!=b  en=off  latency=0  dbl_ovrd=off  block_type=relational
  Relational1 : xbsIndex_r4/Relational  mode=a!=b  en=off  latency=0  dbl_ovrd=off  block_type=relational
  b[0] : xbsIndex_r4/Slice  nbits=1  boolean_output=on  mode=Lower Bit Location + Width  bit1=0  base1=MSB of Input  bit0=0  base0=LSB of Input  dbl_ovrd=off  block_type=slice
  b[1:0] : xbsIndex_r4/Slice  nbits=2  boolean_output=off  mode=Lower Bit Location + Width  bit1=0  base1=MSB of Input  bit0=0  base0=LSB of Input  dbl_ovrd=off  block_type=slice
  b[1] : xbsIndex_r4/Slice  nbits=1  boolean_output=on  mode=Lower Bit Location + Width  bit1=0  base1=MSB of Input  bit0=1  base0=LSB of Input  dbl_ovrd=off  block_type=slice
  b[3] : xbsIndex_r4/Slice  nbits=1  boolean_output=on  mode=Lower Bit Location + Width  bit1=0  base1=MSB of Input  bit0=3  base0=LSB of Input  dbl_ovrd=off  block_type=slice
  b[5:4] : xbsIndex_r4/Slice  nbits=2  boolean_output=off  mode=Lower Bit Location + Width  bit1=0  base1=MSB of Input  bit0=4  base0=LSB of Input  dbl_ovrd=off  block_type=slice
  b[6] : xbsIndex_r4/Slice  nbits=1  boolean_output=on  mode=Lower Bit Location + Width  bit1=0  base1=MSB of Input  bit0=6  base0=LSB of Input  dbl_ovrd=off  block_type=slice
  b[7] : xbsIndex_r4/Slice  nbits=1  boolean_output=on  mode=Lower Bit Location + Width  bit1=0  base1=MSB of Input  bit0=7  base0=LSB of Input  dbl_ovrd=off  block_type=slice
  "b[7] " : xbsIndex_r4/Slice  nbits=1  boolean_output=on  mode=Lower Bit Location + Width  bit1=0  base1=MSB of Input  bit0=7  base0=LSB of Input  dbl_ovrd=off  block_type=slice
  Unsupported : Outport
  wires:
  B3/1 -> b[7]/1
  B6/1 -> b[0]/1, b[1]/1, b[3]/1, b[6]/1, "b[7] "/1, b[5:4]/1
  b[7]/1 -> [CHAN_BW], Logical/1
  b[3]/1 -> [AGGREGATION]
  b[1]/1 -> [NOT_SOUNDING]
  b[0]/1 -> [SMOOTHING]
  b[5:4]/1 -> [STBC], Relational1/1
  b[6]/1 -> [FEC], Logical/2
  "b[7] "/1 -> [SHORT_GI], Logical/3
  B7/1 -> b[1:0]/1
  b[1:0]/1 -> [N_ESS], Relational/1
  Constant/1 -> Relational/2
  Constant1/1 -> Relational1/2
  Relational/1 -> Logical/5
  Relational1/1 -> Logical/4
  Logical/1 -> Unsupported/1

== system wlan_phy_tx_pmd/PSDU Syms Gen/Pkt Data/SIGNAL & HT-SIG Decode/HT-SIG Decode/MCS Decode ==
  note: IEEE 802.11-2012 Table 20-30
      | Single spatial stream 20MHz MCS indexes:
      |
      | 0: BPSK 1/2
      | 1: QPSK 1/2
      | 2: QPSK 3/4
      | 3: 16-QAM 1/2
      | 4: 16-QAM 3/4
      | 5: 64-QAM 2/3
      | 6: 64-QAM 3/4
      | 7: 64-QAM 5/6
      |
      | Mod Order values:
      | 0: BPSK
      | 1: QPSK
      | 2: 16-QAM
      | 3: 64-QAM
      |
      | Code Rate values:
      | 0: 1/2
      | 1: 2/3
      | 2: 3/4
      | 3: 5/6 (HT/VHT only)
      |
      | N_DBPS values:
      | BPSK 1/2: 26
      | QPSK 1/2: 52
      | QPSK 3/4: 78
      | 16-QAM 1/2: 104
      | 16-QAM 3/4: 156
      | 64-QAM 2/3: 208
      | 64-QAM 3/4: 234
      | 64-QAM 5/6: 260
  note: Byte_6[7] = Channel bandwidth (0=20, 1=40)
      | Byte_3[6:0]: MCS (5LSB used here)
  note: % Ouptut word contents:
      | %  b[    0]: Chan bandwidth
      | %  b[ 2: 1]: Num spatial streams
      | %  b[ 4: 3]: Mod order index
      | %  b[ 6: 5]: Code rate index
      | %  b[16: 7]: Coded bits per symbol per stream
      | %  b[26:17]: Data bits per symbol per stream
  note: MCS index values up to 76 are valid. But this block only decodes MCS indexes
      | up to 31. This shortcut is based on observing no use of unequal-modulation
      | MCS indexes in any actual system, and that all UQM schemes were dropped
      | in 802.11ac.
      |
      | I'm technically cheating by calling the UQM MCS indexes invalid. The only real
      | effect of this would be falling back on energy detection for deferring to UQM
      | receptions, since the rate*length block won't attempt a deferral for
      | MCS values declared invalid here.
  note: PHY currently supports MCS 0-7 for BW=20
  B3 : Inport
  B6 : Inport  Port=2
  5LSB : xbsIndex_r4/Slice  nbits=5  boolean_output=off  mode=Lower Bit Location + Width  bit1=0  base1=MSB of Input  bit0=0  base0=LSB of Input  dbl_ovrd=off  block_type=slice
  7LSB : xbsIndex_r4/Slice  nbits=7  boolean_output=off  mode=Lower Bit Location + Width  bit1=0  base1=MSB of Input  bit0=0  base0=LSB of Input  dbl_ovrd=off  block_type=slice
  Concat : xbsIndex_r4/Concat  num_inputs=2  dbl_ovrd=off  block_type=concat
  Constant1 : xbsIndex_r4/Constant  const=76  gui_display_data_type=Fixed-point  arith_type=Unsigned  n_bits=7  bin_pt=0  preci_type=Single  exp_width=8  frac_width=24  explicit_period=off  period=1  equ=P=C  opselect=C  inp2=PCIN>>17  opr=+  inp1=P  carry=CIN  dbl_ovrd=off  block_type=constant
  Constant17 : xbsIndex_r4/Constant  const=7  gui_display_data_type=Fixed-point  arith_type=Unsigned  n_bits=3  bin_pt=0  preci_type=Single  exp_width=8  frac_width=24  explicit_period=off  period=1  equ=P=C  opselect=C  inp2=PCIN>>17  opr=+  inp1=P  carry=CIN  dbl_ovrd=off  block_type=constant
  Constant18 : xbsIndex_r4/Constant  const=31  gui_display_data_type=Fixed-point  arith_type=Unsigned  n_bits=7  bin_pt=0  preci_type=Single  exp_width=8  frac_width=24  explicit_period=off  period=1  equ=P=C  opselect=C  inp2=PCIN>>17  opr=+  inp1=P  carry=CIN  dbl_ovrd=off  block_type=constant
  Convert : xbsIndex_r4/Convert  gui_display_data_type=Boolean  arith_type=Boolean  n_bits=1  bin_pt=0  float_type=Single  exp_bits=8  fraction_bits=24  quantization=Truncate  overflow=Wrap  en=off  latency=0  dbl_ovrd=off  pipeline=off  block_type=convert
  Logical1 : xbsIndex_r4/Logical  logical_function=OR  inputs=2  en=off  latency=0  precision=Full  arith_type=Unsigned  n_bits=16  bin_pt=0  align_bp=on  dbl_ovrd=off  block_type=logical
  ROM : xbsIndex_r4/ROM  depth=numel(mcs_rom_11n)  initVector=mcs_rom_11n  distributed_mem=Block RAM  rst=off  init_reg=0  en=off  latency=1  gui_display_data_type=Fixed-point  arith_type="Signed  (2's comp)"  n_bits=32  bin_pt=0  preci_type=Single  exp_width=8  frac_width=24  dbl_ovrd=off  optimize=Area  use_rpm=on  block_type=sprom
  Relational : xbsIndex_r4/Relational  mode=a>b  en=off  latency=0  dbl_ovrd=off  block_type=relational
  Relational1 : xbsIndex_r4/Relational  mode=a<=b  en=off  latency=0  dbl_ovrd=off  block_type=relational
  b[0] : xbsIndex_r4/Slice  nbits=1  boolean_output=off  mode=Lower Bit Location + Width  bit1=0  base1=MSB of Input  bit0=0  base0=LSB of Input  dbl_ovrd=off  block_type=slice
  b[16:7] : xbsIndex_r4/Slice  nbits=10  boolean_output=off  mode=Lower Bit Location + Width  bit1=0  base1=MSB of Input  bit0=7  base0=LSB of Input  dbl_ovrd=off  block_type=slice
  b[26:17] : xbsIndex_r4/Slice  nbits=10  boolean_output=off  mode=Lower Bit Location + Width  bit1=0  base1=MSB of Input  bit0=17  base0=LSB of Input  dbl_ovrd=off  block_type=slice
  b[2:1] : xbsIndex_r4/Slice  nbits=2  boolean_output=off  mode=Lower Bit Location + Width  bit1=0  base1=MSB of Input  bit0=1  base0=LSB of Input  dbl_ovrd=off  block_type=slice
  b[4:3] : xbsIndex_r4/Slice  nbits=2  boolean_output=off  mode=Lower Bit Location + Width  bit1=0  base1=MSB of Input  bit0=3  base0=LSB of Input  dbl_ovrd=off  block_type=slice
  b[6:5] : xbsIndex_r4/Slice  nbits=2  boolean_output=off  mode=Lower Bit Location + Width  bit1=0  base1=MSB of Input  bit0=5  base0=LSB of Input  dbl_ovrd=off  block_type=slice
  b[7] : xbsIndex_r4/Slice  nbits=1  boolean_output=off  mode=Lower Bit Location + Width  bit1=0  base1=MSB of Input  bit0=7  base0=LSB of Input  dbl_ovrd=off  block_type=slice
  MCS : Outport
  mod_sel : Outport  Port=2
  code_rate : Outport  Port=3
  N_CBPS : Outport  Port=4
  N_DBPS : Outport  Port=5
  N_SS : Outport  Port=6
  Chan_BW : Outport  Port=7
  Unsupported : Outport  Port=8
  MCS Valid : Outport  Port=9
  wires:
  Constant18/1 -> Relational1/2
  Relational1/1 -> MCS Valid/1
  Constant17/1 -> Relational/2
  Relational/1 -> Logical1/2
  B3/1 -> 5LSB/1, 7LSB/1
  B6/1 -> b[7]/1
  ROM/1 -> b[0]/1, b[2:1]/1, b[4:3]/1, b[6:5]/1, b[16:7]/1, b[26:17]/1
  b[7]/1 -> Concat/1
  5LSB/1 -> Concat/2
  Concat/1 -> ROM/1
  7LSB/1 -> MCS/1, Relational/1, Relational1/1
  b[6:5]/1 -> code_rate/1
  b[4:3]/1 -> mod_sel/1
  b[0]/1 -> Chan_BW/1, Convert/1
  b[26:17]/1 -> N_DBPS/1
  b[16:7]/1 -> N_CBPS/1
  b[2:1]/1 -> N_SS/1
  Logical1/1 -> Unsupported/1
  Convert/1 -> Logical1/1

== system wlan_phy_tx_pmd/PSDU Syms Gen/Pkt Data/SIGNAL & HT-SIG Decode/SIGNAL Decode/LENGTH ==
  B0 : Inport
  B1 : Inport  Port=2
  B2 : Inport  Port=3
  1LSB : xbsIndex_r4/Slice  nbits=1  boolean_output=off  mode=Lower Bit Location + Width  bit1=0  base1=MSB of Input  bit0=0  base0=LSB of Input  dbl_ovrd=off  block_type=slice
  3MSB : xbsIndex_r4/Slice  nbits=3  boolean_output=off  mode=Upper Bit Location + Width  bit1=0  base1=MSB of Input  bit0=0  base0=LSB of Input  dbl_ovrd=off  block_type=slice
  Concat : xbsIndex_r4/Concat  num_inputs=3  dbl_ovrd=off  block_type=concat
  Length : Outport
  wires:
  Concat/1 -> Length/1
  1LSB/1 -> Concat/1
  3MSB/1 -> Concat/3
  B1/1 -> Concat/2
  B2/1 -> 1LSB/1
  B0/1 -> 3MSB/1
